simulink model "model_1"  (Simulink 8.7)
settings: Solver=VariableStepAuto  StartTime=0.0  StopTime=1000  RelTol=1e-3
values from neighbouring files (symbols this model uses):
  den_d_f = dict_frac_d_f('denominator')    [simulate_model_debit.m]
  den_d_r = dict_frac_d_r('denominator')    [simulate_model_debit.m]    (also in simulate_model_temperature_pressure.m = dict_d_r_tf('denominator'))
  den_f = dict_frac_f('denominator')    [simulate_model_continuous_debit.m]    (also in simulate_model_debit.m)
  den_r = dict_frac_r('denominator')    [simulate_model_continuous_debit.m]    (also in simulate_model_debit.m)
  num_d_f = dict_frac_d_f('nominator')    [simulate_model_debit.m]
  num_d_r = dict_frac_d_r('nominator')    [simulate_model_debit.m]    (also in simulate_model_temperature_pressure.m = dict_d_r_tf('nominator'))
  num_f = dict_frac_f('nominator')    [simulate_model_continuous_debit.m]    (also in simulate_model_debit.m)
  num_r = dict_frac_r('nominator')    [simulate_model_continuous_debit.m]    (also in simulate_model_debit.m)
  Ts = 0.1    [aist_script.m]    (also in get_rst_regulator.m = dict_perf_criteria('discretisation_period'))
settings Model: Creator=danba  LastModifiedBy=danba
settings DataIOCC: LimitDataPoints=off  SaveFormat=Dataset
settings DebuggingCC: UnderspecifiedInitializationDetection=Simplified  MergeDetectMultiDrivingBlocksExec=error
settings HardwareCC: ProdBitPerPointer=64  ProdLargestAtomicFloat=Float  ProdIntDivRoundTo=Zero  ProdEndianess=LittleEndian  ProdWordSize=64  ProdHWDeviceType=Intel->x86-64 (Windows64)
settings ModelReferenceCC: PropagateSignalLabelsOutOfModel=on
settings ConfigComp: CovModelRefEnable=off

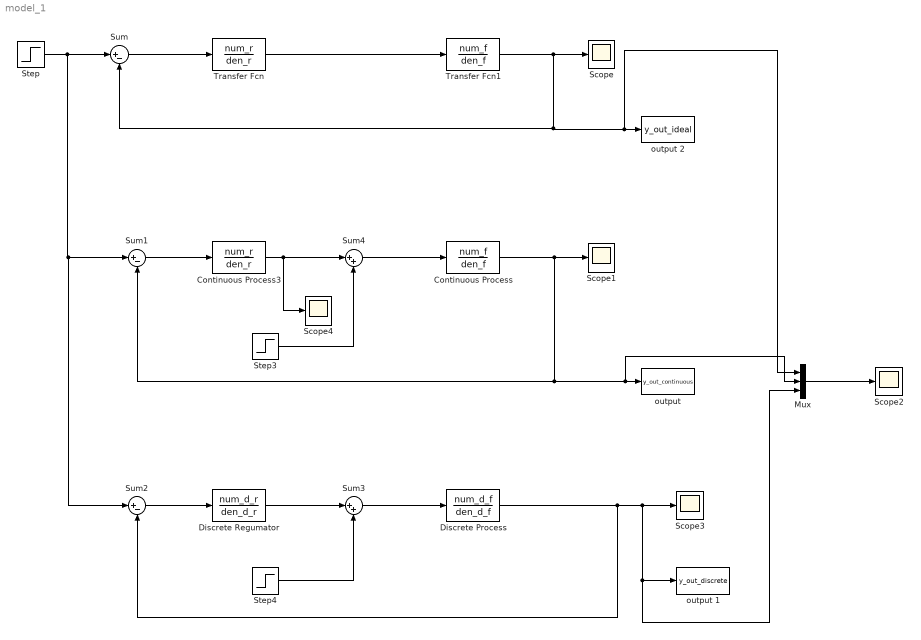
== system model_1 ==
  Continuous Process : TransferFcn  Numerator=num_f  Denominator=den_f
  Continuous Process3 : TransferFcn  Numerator=num_r  Denominator=den_r
  Discrete Process : DiscreteTransferFcn  Numerator=num_d_f  Denominator=den_d_f  SampleTime=Ts
  Discrete Regumator : DiscreteTransferFcn  Numerator=num_d_r  Denominator=den_d_r  SampleTime=Ts  a0EqualsOne=on
  Mux : Mux  Inputs=3
  Scope{,1..4} (5 alike) : Scope
  Step : Step  SampleTime=0.01
  Step3 : Step  Time=3  After=0.2  SampleTime=1
  Step4 : Step  Time=3  After=0.2  SampleTime=1
  Sum : Sum  Inputs=|+-
  Sum1 : Sum  Inputs=|+-
  Sum2 : Sum  Inputs=|+-
  Sum3 : Sum  Inputs=|++
  Sum4 : Sum  Inputs=|++
  Transfer Fcn : TransferFcn  Numerator=num_r  Denominator=den_r
  Transfer Fcn1 : TransferFcn  Numerator=num_f  Denominator=den_f
  "output " : ToWorkspace  VariableName=y_out_continuous  SaveFormat=Structure With Time  SampleTime=-1
  output 1 : ToWorkspace  VariableName=y_out_discrete  SaveFormat=Structure With Time  SampleTime=-1
  output 2 : ToWorkspace  VariableName=y_out_ideal  SaveFormat=Structure With Time  SampleTime=-1
  wires:
  Transfer Fcn/1 -> Transfer Fcn1/1
  Sum/1 -> Transfer Fcn/1
  Transfer Fcn1/1 -> Mux/1, output 2/1, Sum/2, Scope/1
  Continuous Process/1 -> Scope1/1, Mux/2, "output "/1, Sum1/2
  Step/1 -> Sum2/1, Sum1/1, Sum/1
  Sum1/1 -> Continuous Process3/1
  Continuous Process3/1 -> Scope4/1, Sum4/1
  Sum4/1 -> Continuous Process/1
  Step3/1 -> Sum4/2
  Mux/1 -> Scope2/1
  Sum2/1 -> Discrete Regumator/1
  Discrete Process/1 -> output 1/1, Mux/3, Scope3/1, Sum2/2
  Discrete Regumator/1 -> Sum3/1
  Sum3/1 -> Discrete Process/1
  Step4/1 -> Sum3/2
